simulink model "ROPOD_Control_incFlock_UDPTest"  (R2017b)
settings: Solver=ode1  StartTime=0.0  StopTime=Tfinal  FixedStep=Ts  RelTol=1e-3  EnableMultiTasking=on
PreLoadFcn:
  | init_model
InitFcn:
  | init_model
values from neighbouring files (symbols this model uses):
  AgentNumber = 1    [init_model.m]
  FFtheta_intia = 0    [init_model.m]
  FFxy_mass = 0*80    (= 0)    [init_model.m]
  I_fhz_ddelta_cntr = 0    [init_model.m]
  I_fhz_dtheta_cntr = 0.3    [init_model.m]
  I_fhz_dtheta_flock_cntr = 0.1    [init_model.m]
  I_fhz_dvarphi_cntr = 0    [init_model.m]
  I_fhz_dxdy_cntr = 0.25    [init_model.m]
  I_fhz_dxdy_flock_cntr = 0.1    [init_model.m]
  K_gain_ddelta_cntr = 0.1    [init_model.m]
  K_gain_dtheta_cntr = 150    [init_model.m]
  K_gain_dtheta_flock_cntr = 100    [init_model.m]
  K_gain_dvarphi_cntr = 0.05    [init_model.m]
  K_gain_dxdy_cntr = 200    [init_model.m]
  K_gain_dxdy_flock_cntr = 200    [init_model.m]
  LL_wp_fhz_ddelta_cntr = 2    [init_model.m]
  LL_wp_fhz_dtheta_cntr = 20    [init_model.m]
  LL_wp_fhz_dtheta_flock_cntr = 20    [init_model.m]
  LL_wp_fhz_dvarphi_cntr = 10    [init_model.m]
  LL_wp_fhz_dxdy_cntr = 20    [init_model.m]
  LL_wp_fhz_dxdy_flock_cntr = 20    [init_model.m]
  LL_wz_fhz_ddelta_cntr = 2    [init_model.m]
  LL_wz_fhz_dtheta_cntr = 20    [init_model.m]
  LL_wz_fhz_dtheta_flock_cntr = 20    [init_model.m]
  LL_wz_fhz_dvarphi_cntr = 2    [init_model.m]
  LL_wz_fhz_dxdy_cntr = 20    [init_model.m]
  LL_wz_fhz_dxdy_flock_cntr = 20    [init_model.m]
  LPF_fhz_ddelta_cntr = 50    [init_model.m]
  LPF_fhz_ddelta_meas = 50    [init_model.m]
  LPF_fhz_dtheta_cntr = 100    [init_model.m]
  LPF_fhz_dtheta_flock_cntr = 40    [init_model.m]
  LPF_fhz_dvarphi_cntr = 50    [init_model.m]
  LPF_fhz_dvarphi_meas = 50    [init_model.m]
  LPF_fhz_dxdy_cntr = 100    [init_model.m]
  LPF_fhz_dxdy_flock_cntr = 40    [init_model.m]
  max_hw_tau = 7.0    (= 7)    [init_model.m]
  max_ropod_acc_theta = 1.6    [init_model.m]
  max_ropod_acc_xy = 2.0    (= 2)    [init_model.m]
  max_ropod_sw_force = 500    [init_model.m]
  max_ropod_sw_tau = 250    [init_model.m]
  max_ropod_vel_theta = 1.6    [init_model.m]
  max_ropod_vel_xy = 2.0    (= 2)    [init_model.m]
  max_sw_current = 10    [init_model.m]
  Nagents = 2    [init_model.m]
  Nwheels = 4    [Jqwl_numeric_function.m]    (also in S_matrix.m; extract_kinmodel_parameters.m; init_model.m; tau_optimal_dist_vec_fun.m)
  pivot_offs_sws = [0.0243    0.4689    0.3384    5.9050]    [init_model.m]
  ropod_kinmodel_pv = struct2array(ropod_kinmodel_param)    [set_ropod_KinModparams.m]
  ropod_position_inflock = [-1 0 3.1416]    [init_model.m]
  SW_COM1_ENABLE1 = hex2dec('0001')    [init_model.m]
  SW_COM1_ENABLE2 = hex2dec('0002')    [init_model.m]
  SW_COM1_MODE_TORQUE = bitshift(hex2dec('0000'),2)    [init_model.m]
  SW_COM1_MODE_VELOCITY = bitshift(hex2dec('0002'),2)    [init_model.m]
  SW_COM1_USE_TS = hex2dec('8000')    [init_model.m]
  Tinit = 2    [init_model.m]
  Ts = 0.001    [init_model.m]
undefined symbols (not defined in the file or in its folder): DiscIntNeverNeededParam, sw_tau_2_curr
libraries: simulink x61, cstblocks x27, dspsigops x12, dspnetwork x4
(part 5 of 5)

== matlab function ROPOD_Control_incFlock_UDPTest/RopodTorqueDistribution/ROPOD 4SW/ROPOD_4Wheel_sens_own_vel_filter/Glitch removal + LP filter1/Remove_glitches1 ==
  data: vel input; Ts input; encoder input; encoder_out output
function encoder_out  = remove_glitches(vel, Ts, encoder)

persistent last_valid_encoder;
persistent invalid_cnt;

if(isempty(last_valid_encoder))
    last_valid_encoder = encoder;
    invalid_cnt = 0;
end

if abs( (last_valid_encoder-encoder)/Ts ) > 50 % maximum expected velocity rad/sec (2.5 m/s)
    encoder_out = last_valid_encoder + vel*Ts;    
    invalid_cnt = invalid_cnt +1;
else
    encoder_out = encoder;
end

if invalid_cnt>1 
    invalid_cnt = 0;
    encoder_out = encoder;
end

last_valid_encoder = encoder_out;

== matlab function ROPOD_Control_incFlock_UDPTest/RopodTorqueDistribution/ROPOD 4SW/ROPOD_4Wheel_sens_own_vel_filter/Glitch removal + LP filter/Remove_glitches1 ==
  data: vel input; Ts input; encoder input; encoder_out output
function encoder_out  = remove_glitches(vel, Ts, encoder)

persistent last_valid_encoder;
persistent invalid_cnt;

if(isempty(last_valid_encoder))
    last_valid_encoder = encoder;
    invalid_cnt = 0;
end

if abs( (last_valid_encoder-encoder)/Ts ) > 50 % maximum expected velocity rad/sec (2.5 m/s)
    encoder_out = last_valid_encoder + vel*Ts;    
    invalid_cnt = invalid_cnt +1;
else
    encoder_out = encoder;
end

if invalid_cnt>1 
    invalid_cnt = 0;
    encoder_out = encoder;
end

last_valid_encoder = encoder_out;

== matlab function ROPOD_Control_incFlock_UDPTest/RopodTorqueDistribution/ROPOD 4SW/ROPOD_4Wheel_sens_own_vel_filter/Glitch removal + LP filter2/Remove_glitches1 ==
  data: vel input; Ts input; encoder input; encoder_out output
function encoder_out  = remove_glitches(vel, Ts, encoder)

persistent last_valid_encoder;
persistent invalid_cnt;

if(isempty(last_valid_encoder))
    last_valid_encoder = encoder;
    invalid_cnt = 0;
end

if abs( (last_valid_encoder-encoder)/Ts ) > 50 % maximum expected velocity rad/sec (2.5 m/s)
    encoder_out = last_valid_encoder + vel*Ts;    
    invalid_cnt = invalid_cnt +1;
else
    encoder_out = encoder;
end

if invalid_cnt>1 
    invalid_cnt = 0;
    encoder_out = encoder;
end

last_valid_encoder = encoder_out;

== matlab function ROPOD_Control_incFlock_UDPTest/RopodTorqueDistribution/ROPOD 4SW/ROPOD_4Wheel_sens_own_vel_filter/Glitch removal + LP filter3/Remove_glitches1 ==
  data: vel input; Ts input; encoder input; encoder_out output
function encoder_out  = remove_glitches(vel, Ts, encoder)

persistent last_valid_encoder;
persistent invalid_cnt;

if(isempty(last_valid_encoder))
    last_valid_encoder = encoder;
    invalid_cnt = 0;
end

if abs( (last_valid_encoder-encoder)/Ts ) > 50 % maximum expected velocity rad/sec (2.5 m/s)
    encoder_out = last_valid_encoder + vel*Ts;    
    invalid_cnt = invalid_cnt +1;
else
    encoder_out = encoder;
end

if invalid_cnt>1 
    invalid_cnt = 0;
    encoder_out = encoder;
end

last_valid_encoder = encoder_out;

== matlab function ROPOD_Control_incFlock_UDPTest/RopodTorqueDistribution/ROPOD 4SW/ROPOD_4Wheel_sens_own_vel_filter/Glitch removal + LP filter4/Remove_glitches1 ==
  data: vel input; Ts input; encoder input; encoder_out output
function encoder_out  = remove_glitches(vel, Ts, encoder)

persistent last_valid_encoder;
persistent invalid_cnt;

if(isempty(last_valid_encoder))
    last_valid_encoder = encoder;
    invalid_cnt = 0;
end

if abs( (last_valid_encoder-encoder)/Ts ) > 50 % maximum expected velocity rad/sec (2.5 m/s)
    encoder_out = last_valid_encoder + vel*Ts;    
    invalid_cnt = invalid_cnt +1;
else
    encoder_out = encoder;
end

if invalid_cnt>1 
    invalid_cnt = 0;
    encoder_out = encoder;
end

last_valid_encoder = encoder_out;

== matlab function ROPOD_Control_incFlock_UDPTest/RopodProcessWheelSensorData/Odometry and Measurement model 4SW/Jqwl_numeric ==
  data: ropod_kinmodel_param_vec input; v output; delta input; dvarphi input; ena_w input
function v = Jqwl_numeric_wrapper(ropod_kinmodel_param_vec,  delta, dvarphi, ena_w)

v = Jqwl_numeric_function(ropod_kinmodel_param_vec, delta, dvarphi, ena_w);

end

== matlab function ROPOD_Control_incFlock_UDPTest/RopodProcessWheelSensorData/Odometry and Measurement model 4SW/pos_rot_matrix ==
  data: dqr_loc input; theta_odom input; dqr_glb output
function dqr_glb   = zrot(dqr_loc, theta_odom)
%ROPOD_JACOBIAN Summary of this function goes here
%   Detailed explanation goes here


dqr_glb = [  cos(theta_odom) -sin(theta_odom) 0; 
            sin(theta_odom)  cos(theta_odom) 0;
                    0             0  1]*dqr_loc;
end

== matlab function ROPOD_Control_incFlock_UDPTest/RopodVelocityController/platform vel cntr/Inverse Kinematics 4SW/Gl_matrix ==
  data: ropod_kinmodel_param_vec input; Gl output; delta input
function Gl = Gl_matrix_wrapper(ropod_kinmodel_param_vec, delta)

Gl = Gl_matrix_wrapper(ropod_kinmodel_param_vec, delta);

end

== matlab function ROPOD_Control_incFlock_UDPTest/RopodTorqueDistribution/Torque distribution/Gl_matrices ==
  data: ropod_kinmodel_param_vec input; Gl output; delta input; Gtl output; GtSl output
function [Gl, Gtl, GtSl]   = G_matrices( ropod_kinmodel_param_vec, delta)
%ROPOD_JACOBIAN Summary of this function goes here
%   Detailed explanation goes here


Gl    = Gl_matrix_wrapper(ropod_kinmodel_param_vec, delta);
Gtl   = Gl.';
GtSl  = Gtl*S_matrix();
end

== matlab function ROPOD_Control_incFlock_UDPTest/RopodTorqueDistribution/ROPOD 4SW/ROPOD_4Wheel_sens_own_vel_filter/Glitch removal + LP filter5/Remove_glitches1 ==
  data: vel input; Ts input; encoder input; encoder_out output
function encoder_out  = remove_glitches(vel, Ts, encoder)

persistent last_valid_encoder;
persistent invalid_cnt;

if(isempty(last_valid_encoder))
    last_valid_encoder = encoder;
    invalid_cnt = 0;
end

if abs( (last_valid_encoder-encoder)/Ts ) > 50 % maximum expected velocity rad/sec (2.5 m/s)
    encoder_out = last_valid_encoder + vel*Ts;    
    invalid_cnt = invalid_cnt +1;
else
    encoder_out = encoder;
end

if invalid_cnt>1 
    invalid_cnt = 0;
    encoder_out = encoder;
end

last_valid_encoder = encoder_out;

== matlab function ROPOD_Control_incFlock_UDPTest/RopodTorqueDistribution/Torque distribution/platform_forces_2_tau_dist_optimal ==
  data: GtSl input; taubody input; ena_w input; Ttaud output; tau_max input; taubody_sc output
function [Ttaud, taubody_sc]   = Ttaud_optimal_vec( GtSl, taubody, ena_w , tau_max)
%#codegen

[Ttaud, taubody_sc]   = tau_optimal_dist_vec_fun( GtSl, taubody, ena_w, tau_max);

end

== matlab function ROPOD_Control_incFlock_UDPTest/From ROS (Parameters and topics)/rot_matrix2 ==
  data: dqr_glb input; theta input; dqr_loc output
function dqr_loc   = zrot(dqr_glb, theta)
%ROPOD_JACOBIAN Summary of this function goes here
%   Detailed explanation goes here


dqr_loc = [  cos(-theta) -sin(-theta) 0; 
            sin(-theta)  cos(-theta) 0;
                    0             0  1]*dqr_glb;
end

== matlab function ROPOD_Control_incFlock_UDPTest/RopodTorqueDistribution/ROPOD 4SW/ROPOD_4Wheel_sens_own_vel_filter/Glitch removal + LP filter6/Remove_glitches1 ==
  data: vel input; Ts input; encoder input; encoder_out output
function encoder_out  = remove_glitches(vel, Ts, encoder)

persistent last_valid_encoder;
persistent invalid_cnt;

if(isempty(last_valid_encoder))
    last_valid_encoder = encoder;
    invalid_cnt = 0;
end

if abs( (last_valid_encoder-encoder)/Ts ) > 50 % maximum expected velocity rad/sec (2.5 m/s)
    encoder_out = last_valid_encoder + vel*Ts;    
    invalid_cnt = invalid_cnt +1;
else
    encoder_out = encoder;
end

if invalid_cnt>1 
    invalid_cnt = 0;
    encoder_out = encoder;
end

last_valid_encoder = encoder_out;

== matlab function ROPOD_Control_incFlock_UDPTest/RopodTorqueDistribution/ROPOD 4SW/ROPOD_4Wheel_sens_own_vel_filter/Glitch removal + LP filter7/Remove_glitches1 ==
  data: vel input; Ts input; encoder input; encoder_out output
function encoder_out  = remove_glitches(vel, Ts, encoder)

persistent last_valid_encoder;
persistent invalid_cnt;

if(isempty(last_valid_encoder))
    last_valid_encoder = encoder;
    invalid_cnt = 0;
end

if abs( (last_valid_encoder-encoder)/Ts ) > 50 % maximum expected velocity rad/sec (2.5 m/s)
    encoder_out = last_valid_encoder + vel*Ts;    
    invalid_cnt = invalid_cnt +1;
else
    encoder_out = encoder;
end

if invalid_cnt>1 
    invalid_cnt = 0;
    encoder_out = encoder;
end

last_valid_encoder = encoder_out;

== matlab function ROPOD_Control_incFlock_UDPTest/RopodTorqueDistribution/ROPOD 4SW/ROPOD_4Wheel_sens_own_vel_filter/Glitch removal + LP filter8/Remove_glitches1 ==
  data: vel input; Ts input; encoder input; encoder_out output
function encoder_out  = remove_glitches(vel, Ts, encoder)

persistent last_valid_encoder;
persistent invalid_cnt;

if(isempty(last_valid_encoder))
    last_valid_encoder = encoder;
    invalid_cnt = 0;
end

if abs( (last_valid_encoder-encoder)/Ts ) > 50 % maximum expected velocity rad/sec (2.5 m/s)
    encoder_out = last_valid_encoder + vel*Ts;    
    invalid_cnt = invalid_cnt +1;
else
    encoder_out = encoder;
end

if invalid_cnt>1 
    invalid_cnt = 0;
    encoder_out = encoder;
end

last_valid_encoder = encoder_out;

== matlab function ROPOD_Control_incFlock_UDPTest/RopodTorqueDistribution/ROPOD 4SW/ROPOD_4Wheel_sens_own_vel_filter/Glitch removal + LP filter10/Remove_glitches1 ==
  data: vel input; Ts input; encoder input; encoder_out output
function encoder_out  = remove_glitches(vel, Ts, encoder)

persistent last_valid_encoder;
persistent invalid_cnt;

if(isempty(last_valid_encoder))
    last_valid_encoder = encoder;
    invalid_cnt = 0;
end

if abs( (last_valid_encoder-encoder)/Ts ) > 50 % maximum expected velocity rad/sec (2.5 m/s)
    encoder_out = last_valid_encoder + vel*Ts;    
    invalid_cnt = invalid_cnt +1;
else
    encoder_out = encoder;
end

if invalid_cnt>1 
    invalid_cnt = 0;
    encoder_out = encoder;
end

last_valid_encoder = encoder_out;

== matlab function ROPOD_Control_incFlock_UDPTest/RopodTorqueDistribution/ROPOD 4SW/ROPOD_4Wheel_sens_own_vel_filter/Glitch removal + LP filter11/Remove_glitches1 ==
  data: vel input; Ts input; encoder input; encoder_out output
function encoder_out  = remove_glitches(vel, Ts, encoder)

persistent last_valid_encoder;
persistent invalid_cnt;

if(isempty(last_valid_encoder))
    last_valid_encoder = encoder;
    invalid_cnt = 0;
end

if abs( (last_valid_encoder-encoder)/Ts ) > 50 % maximum expected velocity rad/sec (2.5 m/s)
    encoder_out = last_valid_encoder + vel*Ts;    
    invalid_cnt = invalid_cnt +1;
else
    encoder_out = encoder;
end

if invalid_cnt>1 
    invalid_cnt = 0;
    encoder_out = encoder;
end

last_valid_encoder = encoder_out;

== matlab function ROPOD_Control_incFlock_UDPTest/RopodTorqueDistribution/ROPOD 4SW/ROPOD_4Wheel_sens_own_vel_filter/Glitch removal + LP filter9/Remove_glitches1 ==
  data: vel input; Ts input; encoder input; encoder_out output
function encoder_out  = remove_glitches(vel, Ts, encoder)

persistent last_valid_encoder;
persistent invalid_cnt;

if(isempty(last_valid_encoder))
    last_valid_encoder = encoder;
    invalid_cnt = 0;
end

if abs( (last_valid_encoder-encoder)/Ts ) > 50 % maximum expected velocity rad/sec (2.5 m/s)
    encoder_out = last_valid_encoder + vel*Ts;    
    invalid_cnt = invalid_cnt +1;
else
    encoder_out = encoder;
end

if invalid_cnt>1 
    invalid_cnt = 0;
    encoder_out = encoder;
end

last_valid_encoder = encoder_out;

== matlab function ROPOD_Control_incFlock_UDPTest/MATLAB Function2 ==
  data: gamepad_input input; force_out output; max_force input
function force_out = fcn(gamepad_input, max_force)

switch gamepad_input
    case 1
        force_out = [0 max_force 0]';
    case 2
        force_out = [0 -max_force 0]';
    case 3
        force_out = [-max_force 0 0]';
    case 4
        force_out = [max_force 0 0]';
    otherwise
        force_out = [0 0 0]';

end

== matlab function ROPOD_Control_incFlock_UDPTest/RopodVelocityController1/Deserialization ==
  data: ext_agents_configuration input; enable_ext_agents output; position_ext_agents output; constraints_ext_agents output
function [enable_ext_agents, position_ext_agents, constraints_ext_agents ] = deserializeFlockData(ext_agents_configuration)

size_pa = 12;
Nagents = (length(ext_agents_configuration)/size_pa) + 1; %

enable_ext_agents = zeros(1,Nagents-1);
position_ext_agents = zeros(3,Nagents-1);
constraints_ext_agents = zeros(4*2,Nagents-1);

for i_cnt = 1:(Nagents-1)
    enable_ext_agents(i_cnt) = ext_agents_configuration((Nagents-1)*(i_cnt-1)+1);
    position_ext_agents(:,i_cnt) = ext_agents_configuration((Nagents-1)*(i_cnt-1)+(2:4));
    constraints_ext_agents(:,i_cnt) = ext_agents_configuration((Nagents-1)*(i_cnt-1)+(5:size_pa));
end

== matlab function ROPOD_Control_incFlock_UDPTest/RopodVelocityController1/Optimization Matrices Calculation ==
  data: enable_agents input; A_agents output; AR_agents output; bR_agents output; position_agents input; constraints_agents input
function [A_agents, AR_agents, bR_agents] = computeOptMatrices(enable_agents, position_agents, constraints_agents )

Nagents = length(enable_agents); %

A_agents = zeros(3,3,Nagents);
AR_agents = zeros(6,3,Nagents); % TODO: 4 lines +2 of ropods
bR_agents = zeros(6,1,Nagents);

for i_agnt = 1:Nagents
    x_agnt = position_agents(1,i_agnt);
    x_agnt_torque = x_agnt;
    y_agnt = position_agents(2,i_agnt);
    y_agnt_torque = y_agnt;
    th_agnt = position_agents(3,i_agnt);
    
    % For now no torque is assigned to ropods.
    % On one hand it is not desired, on the other,
    % when arm aproaches 0, more torque is assigned and
    % there is a singularity
    tau_max_ropod = 0;
    if (x_agnt_torque==0)
        x_agnt_torque = 0.1;
    elseif(abs(x_agnt_torque) < 0.1)
        x_agnt_torque = 0.1*sign(x_agnt_torque);
    end
    
    if (y_agnt_torque==0)
        y_agnt_torque = 0.1;
    elseif(abs(y_agnt_torque) < 0.1)
        y_agnt_torque = 0.1*sign(y_agnt_torque);
    end    
    
    A_agents(:,:,i_agnt) = ...
        [
                                          cos(th_agnt)                                    sin(th_agnt)    1/y_agnt_torque;
                                          sin(th_agnt)                                    cos(th_agnt)   -1/x_agnt_torque;
        -( y_agnt*cos(th_agnt) + x_agnt*sin(th_agnt) )   ( x_agnt*cos(th_agnt) - y_agnt*sin(th_agnt) )           1;
        ];
    
    
   
    AgntConst = zeros(4,2);
    for i_agcnst = 1:4 % constraints of a single agent
        AgntConst(i_agcnst,:) = constraints_agents(2*(i_agcnst-1)+1 : 2*(i_agcnst-1)+2 ,i_agnt);      
    end

    AR_agents(:,:,i_agnt) = ...
        [
        [AgntConst(1,2)-AgntConst(2,2) AgntConst(2,1)-AgntConst(1,1) 0];
        [AgntConst(2,2)-AgntConst(3,2) AgntConst(3,1)-AgntConst(2,1) 0];
        [AgntConst(3,2)-AgntConst(4,2) AgntConst(4,1)-AgntConst(3,1) 0];
        [AgntConst(4,2)-AgntConst(1,2) AgntConst(1,1)-AgntConst(4,1) 0];
        [0 0 1];
        [0 0 -1];
        ];
    % prevent trivial problem leading to incorrect solution
    if(AR_agents(1:4,:,i_agnt) ==  zeros(4,3))
        small_number = 0.1;
        AR_agents(1:4,:,i_agnt) =   [   -small_number -small_number 0;
                                         small_number -small_number 0;
                                         small_number  small_number 0;
                                        -small_number  small_number 0;
                                    ];                 
    end
    
    bR_agents(:,:,i_agnt) = ...
        [
        -(AgntConst(1,1)*AgntConst(2,2)-AgntConst(2,1)*AgntConst(1,2));
        -(AgntConst(2,1)*AgntConst(3,2)-AgntConst(3,1)*AgntConst(2,2));
        -(AgntConst(3,1)*AgntConst(4,2)-AgntConst(4,1)*AgntConst(3,2));
        -(AgntConst(4,1)*AgntConst(1,2)-AgntConst(1,1)*AgntConst(4,2));
        -tau_max_ropod;
        -tau_max_ropod; 
        ];
end

== matlab function ROPOD_Control_incFlock_UDPTest/MATLAB Function ==
  data: ext_agents_configuration_ini input; out_ext_agents_configuration output; message_in input; length_in input
function out_ext_agents_configuration = concatenate_agents_conf(ext_agents_configuration_ini, message_in, length_in)
size_ag_conf = 1+3+8;
Nagents = length(ext_agents_configuration_ini)/size_ag_conf +1;
% ext_agents_configuration_ini(1) - enabled
% ext_agents_configuration_ini(2:4) - position
% ext_agents_configuration_ini(5:12) - 4 constraints points

% message_in(1) - agentNumber. By definition is from 2 to Nagents. 1 is reserved for coordinator
% message_in(2:end) - agent configuration

persistent ext_agents_configuration
if isempty(ext_agents_configuration)
    ext_agents_configuration = ext_agents_configuration_ini;
end

agentNumber = message_in(1);
if(length_in==size_ag_conf && agentNumber>=2 && agentNumber<=Nagents)
    i_agnt = agentNumber-1;
    ext_agents_configuration( (i_agnt-1)*size_ag_conf+2 : i_agnt*size_ag_conf) = message_in(2:end);
end


out_ext_agents_configuration = ext_agents_configuration;




end

== matlab function ROPOD_Control_incFlock_UDPTest/RopodVelocityController1/Own Constrainst Calculator ==
  data: enable_local_robot output; ropod_kinmodel_param_vec input; flock_control_mode input; tau_max input; constraints_local_robot output; ena_sw input
function [enable_local_robot, constraints_local_robot ] = calculateConstraints(ropod_kinmodel_param_vec, flock_control_mode, tau_max, ena_sw)
Nwheels = length(ena_sw);

[  rW1_1,rW1_2,rW1_3,rW1_4,rW2_1,rW2_2,rW2_3,rW2_4,...
    s_w,...
    d_w, ...
    CW1_1,CW1_2,CW1_3,CW1_4,CW2_1,CW2_2,CW2_3,CW2_4 ...
    ]= extract_kinmodel_parameters(ropod_kinmodel_param_vec);

rw = rW1_1;
% Conservtaive approach use only forward force of smartwheel, which is
% the smallest of all directions. In any case forces in other directions
% last little since the wheels will align in the direction of movement.

Fsw_max = 2*tau_max/rw;


CW = [[CW1_1 ; CW2_1], [CW1_2 ; CW2_2], [CW1_3 ; CW2_3], [CW1_4 ; CW2_4]];


%% First compute the matrix from v to W_wh

% Gi = zeros([2 3]);
G = zeros(2*Nwheels,3);
M = zeros(2*Nwheels,2*Nwheels);

for i=1:Nwheels    
    % To obtain pivot velocities in Robot coordinates, add vectors of
    % translations and movement due to angular velocity.
    Gi = [1 0 -CW(2,i);
                 0 1  CW(1,i)];             
    
    G(2*i-1:2*i,:) = Gi;    
    M(2*i-1:2*i,2*i-1:2*i)=diag([ena_sw(i) ena_sw(i)]);
end     

GtS = (M*G)'*eye(8);

if(flock_control_mode==0 || sum(ena_sw)<2)
    enable_local_robot = 0;
    Fx_max_ropod = 0;
    Fy_max_ropod = 0;    
else
    enable_local_robot = 1;
    % Compute Force at pivots to actuate 1N in x at the ropod. Then scale up.
    Fpiv1Nx = pinv(GtS)*[1 0 0]';
    Fx_max_ropod = Fsw_max/max(abs(Fpiv1Nx));
    Fpiv1Ny = pinv(GtS)*[0 1 0]';
    Fy_max_ropod = Fsw_max/max(abs(Fpiv1Ny));    
end


% Eight elements with x,y position of constraint
constraints_local_robot = ...
    [
    Fx_max_ropod,   0, ...
    0,              Fy_max_ropod , ...
    -Fx_max_ropod,  0, ...
    0,             -Fy_max_ropod  ...
    ]';

end

== matlab function ROPOD_Control_incFlock_UDPTest/MATLAB Function1 ==
  data: AgentNumber input; WrenchAgent output; message_in input; length_msg input
function WrenchAgent = concatenate_agents_conf(AgentNumber, message_in, length_msg)
Nagents = length(message_in)/3;

persistent WrenchAgent_

if isempty(WrenchAgent_)
    WrenchAgent_ = [0 0 0]';
end

if ( length_msg == (3*Nagents) && AgentNumber<=Nagents)
    WrenchAgent_ = message_in((AgentNumber-1)*3+1:(AgentNumber-1)*3+3);
end

WrenchAgent = WrenchAgent_;



end

== matlab function ROPOD_Control_incFlock_UDPTest/RopodVelocityController1/Wrench Distributor ==
  data: wact input; is_coordinator input; Arow input; AR input; bR input; wR1 output; w_agents output; alpha output
function [wR1, w_agents, alpha] = DistributeWrenchOptimally(wact, is_coordinator, Arow, AR, bR)
%#codegen

Nagents = size(AR,3);
    if is_coordinator == 1  
        %% Function initalization
        % x = [wR1; ...; wRi; alpha]
        % wact = [Fx; Fy; \tau_z]
       
    %     useAlpha = 1;
    %     if useAlpha == 1
        %% Equalities
        Aeq = [zeros(3,3*Nagents) wact];
        beq = wact;
        % Aeq and beq might  be extended to include alpha ? (For which there no
        % equalities)

        %% Inequalities  
        A = zeros(2*(3*Nagents+1), Nagents*3+1);
        b = zeros(2*(3*Nagents+1), 1);

        % Put inequalities of each ropod into the master optimizer
        for iagent = 1:Nagents
            Aeq(:, 3*(iagent-1)+1:3*(iagent-1)+3) = Arow(:,:,iagent);
            A(6*(iagent-1)+1:6*(iagent-1)+6  ,  3*(iagent-1)+1:3*(iagent-1)+3) = AR(:,:,iagent);
            b(6*(iagent-1)+1:6*(iagent-1)+6) = bR(:,:,iagent);
        end
        
%         A(1:6, 1:3) = AR1;
%         b(1:6) = bR1;
%         
%         if Nagents == 2
%             A(7:12, 4:6) = AR2; % For 2 ropods
%             b(7:12) = bR2;
%         end

        % Inequalities for alpha
        A((Nagents*6)+1:(Nagents*6)+2, 3*Nagents+1) = [1; -1];
        b((Nagents*6)+1:(Nagents*6)+2) = [0; -1];

        H = eye(3*Nagents+1);
        H(3*Nagents+1, 3*Nagents+1) = 1;
        % Find the lower-triangular Cholesky decomposition of H.

        % We assume diagonal and square H;
        Linv = zeros(3*Nagents+1); 
        for icnt = 1:(3*Nagents+1)
            Linv(icnt,icnt) = 1/H(icnt,icnt); % equivalent to H = P^2H
        end        
        
    %     Linv = eye(3*Nagents+1);
        f = zeros(3*Nagents+1, 1);
        Fxmax = 425;
        Fymax = 1700;
        f(3*Nagents+1) = 0.5*(Fxmax^2+Fymax^2);
        x = zeros(3*Nagents+1,1);
        status = 0;
%         [x, status] = mpcqpsolver(Linv, f, A, b, Aeq, beq, false(Nagents*6+2, 1), mpcqpsolverOptions());
        [x, status] = mpcqpsolver(Linv, f, A, b, Aeq, beq, false(2*(3*Nagents+1), 1), mpcqpsolverOptions());
        if status <= 0
%             disp('Problem is not feasible!');
              wR1 = zeros(3,1);
              w_agents = zeros(3*(Nagents-1), 1);
              alpha = 1;
        else
            wR1 = x(1:3);
            if Nagents == 1
                w_agents = zeros(3, 1);
            else
                w_agents = x(4:Nagents*3);
            end
            alpha = x(Nagents*3 + 1);            
        end

    else
        wR1 = wact;
        w_agents = zeros(3*(Nagents-1), 1);
        alpha = 0;
    end
end

== matlab function ROPOD_Control_incFlock_UDPTest/RopodTorqueDistribution/wheel flip compensation/MATLAB Function ==
  data: tl input; tl_out output; tr input; ropod_kinmodel_param_vec input size=18; tr_out output; kmax input; sc output
function [tl_out,tr_out, sc] = fcn(tl, tr, ropod_kinmodel_param_vec, kmax)

[  rW1_1,rW1_2,rW1_3,rW1_4,rW2_1,rW2_2,rW2_3,rW2_4,...
    s_w,...
    d_w, ...
    CW1_1,CW1_2,CW1_3,CW1_4,CW2_1,CW2_2,CW2_3,CW2_4 ...
    ]= extract_kinmodel_parameters(ropod_kinmodel_param_vec);

Fxi = (tl/rW1_1+tr/rW1_2);
Fyi = (tr/rW1_2-tl/rW1_1)*(d_w/(2*s_w));
theta = atan2(Fyi,Fxi);

Fsize = sqrt(Fxi*Fxi+Fyi*Fyi);
if Fsize> 30
   sc = (1+(kmax-1)*abs(sin(theta)));
else
    sc = 1;
end

tl_out = tl*sc;
tr_out = tr*sc;

== matlab function ROPOD_Control_incFlock_UDPTest/RopodTorqueDistribution/wheel flip compensation/MATLAB Function1 ==
  data: tl input; tl_out output; tr input; ropod_kinmodel_param_vec input size=18; tr_out output; kmax input
function [tl_out,tr_out] = fcn(tl, tr, ropod_kinmodel_param_vec, kmax)

[  rW1_1,rW1_2,rW1_3,rW1_4,rW2_1,rW2_2,rW2_3,rW2_4,...
    s_w,...
    d_w, ...
    CW1_1,CW1_2,CW1_3,CW1_4,CW2_1,CW2_2,CW2_3,CW2_4 ...
    ]= extract_kinmodel_parameters(ropod_kinmodel_param_vec);

Fxi = (tl/rW1_1+tr/rW1_2);
Fyi = (tr/rW1_2-tl/rW1_1)*(d_w/(2*s_w));
theta = atan2(Fyi,Fxi);

Fsize = sqrt(Fxi*Fxi+Fyi*Fyi);
if Fsize> 30
   sc = (1+(kmax-1)*abs(sin(theta)));
else
    sc = 1;
end

tl_out = tl*sc;
tr_out = tr*sc;

== matlab function ROPOD_Control_incFlock_UDPTest/RopodTorqueDistribution/wheel flip compensation/MATLAB Function2 ==
  data: tl input; tl_out output; tr input; ropod_kinmodel_param_vec input size=18; tr_out output; kmax input
function [tl_out,tr_out] = fcn(tl, tr, ropod_kinmodel_param_vec, kmax)

[  rW1_1,rW1_2,rW1_3,rW1_4,rW2_1,rW2_2,rW2_3,rW2_4,...
    s_w,...
    d_w, ...
    CW1_1,CW1_2,CW1_3,CW1_4,CW2_1,CW2_2,CW2_3,CW2_4 ...
    ]= extract_kinmodel_parameters(ropod_kinmodel_param_vec);

Fxi = (tl/rW1_1+tr/rW1_2);
Fyi = (tr/rW1_2-tl/rW1_1)*(d_w/(2*s_w));
theta = atan2(Fyi,Fxi);

Fsize = sqrt(Fxi*Fxi+Fyi*Fyi);
if Fsize> 30
   sc = (1+(kmax-1)*abs(sin(theta)));
else
    sc = 1;
end

tl_out = tl*sc;
tr_out = tr*sc;

== matlab function ROPOD_Control_incFlock_UDPTest/RopodTorqueDistribution/wheel flip compensation/MATLAB Function3 ==
  data: tl input; tl_out output; tr input; ropod_kinmodel_param_vec input size=18; tr_out output; kmax input
function [tl_out,tr_out] = fcn(tl, tr, ropod_kinmodel_param_vec, kmax)

[  rW1_1,rW1_2,rW1_3,rW1_4,rW2_1,rW2_2,rW2_3,rW2_4,...
    s_w,...
    d_w, ...
    CW1_1,CW1_2,CW1_3,CW1_4,CW2_1,CW2_2,CW2_3,CW2_4 ...
    ]= extract_kinmodel_parameters(ropod_kinmodel_param_vec);

Fxi = (tl/rW1_1+tr/rW1_2);
Fyi = (tr/rW1_2-tl/rW1_1)*(d_w/(2*s_w));
theta = atan2(Fyi,Fxi);

Fsize = sqrt(Fxi*Fxi+Fyi*Fyi);
if Fsize> 30
   sc = (1+(kmax-1)*abs(sin(theta)));
else
    sc = 1;
end

tl_out = tl*sc;
tr_out = tr*sc;
